simulink model "zad1_repr_graf_niel_dyn_mod_ciagly"  (R2014b)
settings: Solver=ode45  StartTime=0.0  StopTime=100  RelTol=1e-3
values from neighbouring files (symbols this model uses):
  a1 = 0.39    [dane_poczatkowe.mat]
  a2 = 0.45    [dane_poczatkowe.mat]
  a3 = -2.91    [dane_poczatkowe.mat]
  a4 = 0.25    [dane_poczatkowe.mat]
  K = 3.5    [dane_poczatkowe.mat]
  T1 = 5    [dane_poczatkowe.mat]
  T2 = 9    [dane_poczatkowe.mat]
  x1 = 0    [dane_poczatkowe.mat]
  x2 = 0    [dane_poczatkowe.mat]
settings Model: Creator=Konrad  LastModifiedBy=Konrad

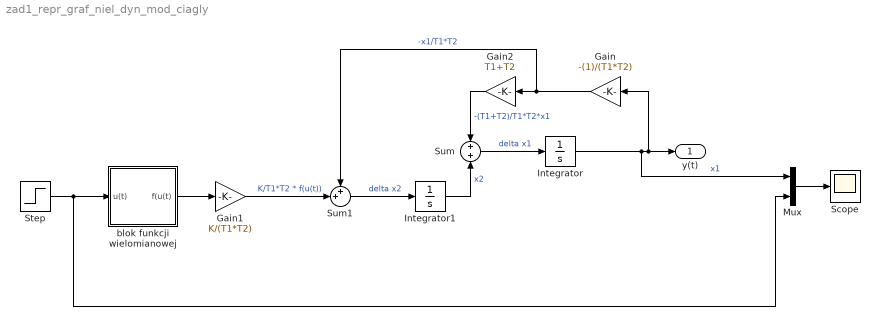
== system zad1_repr_graf_niel_dyn_mod_ciagly ==
  Gain : Gain  Gain=-(1)/(T1*T2)
  Gain1 : Gain  Gain=K/(T1*T2)
  Gain2 : Gain  Gain=T1+T2
  Integrator : Integrator  InitialCondition=x1  ContinuousStateAttributes='x1'
  Integrator1 : Integrator  InitialCondition=x2  ContinuousStateAttributes='x2'
  Mux : Mux  Inputs=2
  Scope : Scope
  Step : Step  SampleTime=0
  Sum : Sum
  Sum1 : Sum  Inputs=++|
  blok funkcji wielomianowej : Subsystem
  y(t) : Outport
  wires:
  Integrator/1 -> Mux/1, Gain/1, y(t)/1  "x1"
  Sum/1 -> Integrator/1  "delta x1"
  Integrator1/1 -> Sum/2  "x2"
  Gain/1 -> Sum1/1, Gain2/1  "-x1/T1*T2"
  Gain2/1 -> Sum/1  "-(T1+T2)/T1*T2*x1"
  Sum1/1 -> Integrator1/1  "delta x2"
  Gain1/1 -> Sum1/2  "K/T1*T2 * f(u(t))"
  blok funkcji wielomianowej/1(f(u(t)) -> Gain1/1
  Step/1 -> Mux/2, blok funkcji wielomianowej/1(u(t))
  Mux/1 -> Scope/1

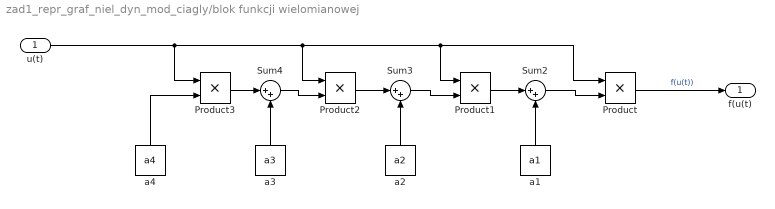
== system zad1_repr_graf_niel_dyn_mod_ciagly/blok funkcji wielomianowej ==
  u(t) : Inport
  Product{,1..3} (4 alike) : Product
  Sum2 : Sum  Inputs=|++
  Sum3 : Sum  Inputs=|++
  Sum4 : Sum  Inputs=|++
  a1 : Constant  Value=a1
  a2 : Constant  Value=a2
  a3 : Constant  Value=a3
  a4 : Constant  Value=a4
  f(u(t) : Outport
  wires:
  u(t)/1 -> Product/1, Product1/1, Product2/1, Product3/1
  Product1/1 -> Sum2/1
  Product2/1 -> Sum3/1
  Sum2/1 -> Product/2
  Product/1 -> f(u(t)/1  "f(u(t))"
  Product3/1 -> Sum4/1
  a1/1 -> Sum2/2
  a2/1 -> Sum3/2
  Sum3/1 -> Product1/2
  a3/1 -> Sum4/2
  Sum4/1 -> Product2/2
  a4/1 -> Product3/2
